simulink model "model"  (R2023a)
settings: Solver=ode4  StartTime=0.0  StopTime=15  FixedStep=0.002  RelTol=1e-3
InitFcn:
  | init;
undefined symbols (not defined in the file): g, N, T, t_f, v_c
libraries: dspsrcs4 x1
settings Model: Creator=Ali  LastModifiedBy=Ali

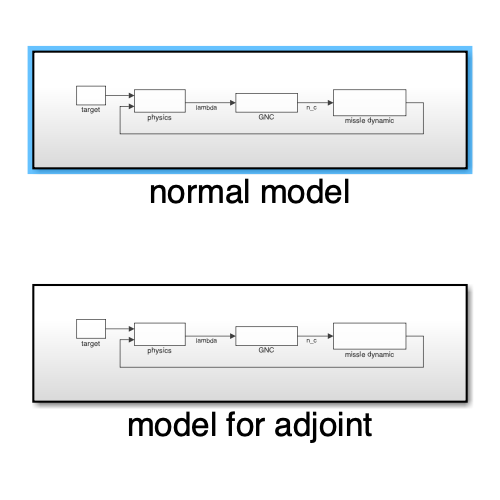
[thumbnail: Simulink's stored preview of the top-level diagram]
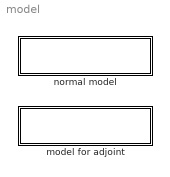
== system model ==
  model for adjoint : Subsystem
  normal model : Subsystem

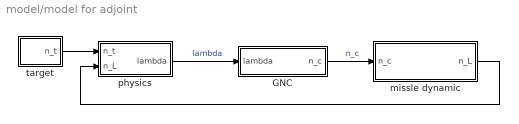
== system model/model for adjoint ==
  GNC : Subsystem
  missle dynamic : Subsystem
  physics : Subsystem
  target : Subsystem
  wires:
  physics/1(lambda) -> GNC/1(lambda)  "lambda"
  target/1(n_t) -> physics/1(n_t)
  GNC/1(n_c) -> missle dynamic/1(n_c)  "n_c"
  missle dynamic/1(n_L) -> physics/2(n_L)

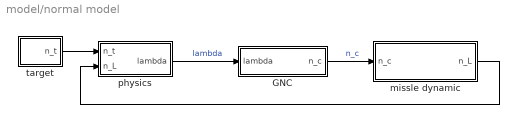
== system model/normal model ==
  GNC : Subsystem
  missle dynamic : Subsystem
  physics : Subsystem
  target : Subsystem
  wires:
  physics/1(lambda) -> GNC/1(lambda)  "lambda"
  target/1(n_t) -> physics/1(n_t)
  GNC/1(n_c) -> missle dynamic/1(n_c)  "n_c"
  missle dynamic/1(n_L) -> physics/2(n_L)

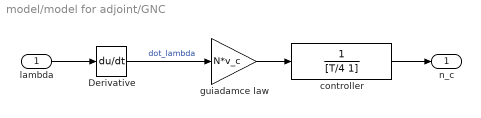
== system model/model for adjoint/GNC ==
  lambda : Inport
  Derivative : Derivative
  controller : TransferFcn  Denominator=[T/4 1]
  guiadamce law : Gain  Gain=N*v_c
  n_c : Outport
  wires:
  guiadamce law/1 -> controller/1
  lambda/1 -> Derivative/1
  Derivative/1 -> guiadamce law/1  "dot_lambda"
  controller/1 -> n_c/1

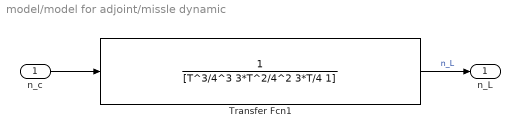
== system model/model for adjoint/missle dynamic ==
  n_c : Inport
  Transfer Fcn1 : TransferFcn  Denominator=[T^3/4^3 3*T^2/4^2 3*T/4 1]
  n_L : Outport
  wires:
  Transfer Fcn1/1 -> n_L/1  "n_L"
  n_c/1 -> Transfer Fcn1/1

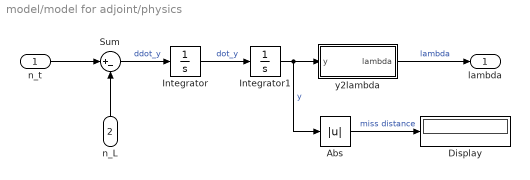
== system model/model for adjoint/physics ==
  n_t : Inport
  n_L : Inport  Port=2
  Abs : Abs  SaturateOnIntegerOverflow=off
  Display : Display
  Integrator : Integrator
  Integrator1 : Integrator
  Sum : Sum  Inputs=|+-
  y2lambda : Subsystem
  lambda : Outport
  wires:
  Sum/1 -> Integrator/1  "ddot_y"
  n_t/1 -> Sum/1
  n_L/1 -> Sum/2
  y2lambda/1(lambda) -> lambda/1  "lambda"
  Integrator/1 -> Integrator1/1  "dot_y"
  Integrator1/1 -> Abs/1, y2lambda/1(y)  "y"
  Abs/1 -> Display/1  "miss distance"

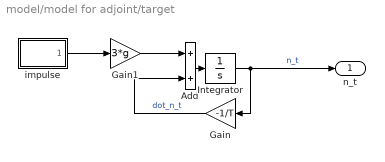
== system model/model for adjoint/target ==
  Add : Sum
  Gain : Gain  Gain=-1/T
  Gain1 : Gain  Gain=3*g
  Integrator : Integrator
  impulse : Subsystem
  n_t : Outport
  wires:
  Gain/1 -> Add/2  "dot_n_t"
  Integrator/1 -> Gain/1, n_t/1  "n_t"
  impulse/1(impulse) -> Gain1/1
  Gain1/1 -> Add/1
  Add/1 -> Integrator/1

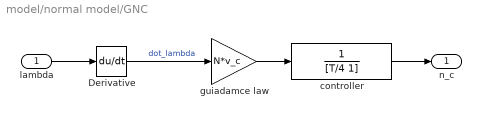
== system model/normal model/GNC ==
  lambda : Inport
  Derivative : Derivative
  controller : TransferFcn  Denominator=[T/4 1]
  guiadamce law : Gain  Gain=N*v_c
  n_c : Outport
  wires:
  guiadamce law/1 -> controller/1
  lambda/1 -> Derivative/1
  Derivative/1 -> guiadamce law/1  "dot_lambda"
  controller/1 -> n_c/1

== system model/normal model/missle dynamic ==
  n_c : Inport
  Transfer Fcn1 : TransferFcn  Denominator=[T^3/4^3 3*T^2/4^2 3*T/4 1]
  n_L : Outport
  wires:
  Transfer Fcn1/1 -> n_L/1  "n_L"
  n_c/1 -> Transfer Fcn1/1

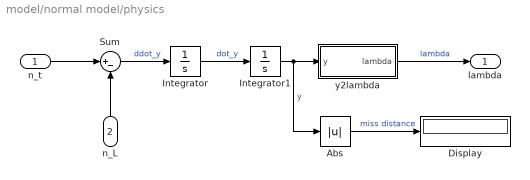
== system model/normal model/physics ==
  n_t : Inport
  n_L : Inport  Port=2
  Abs : Abs  SaturateOnIntegerOverflow=off
  Display : Display
  Integrator : Integrator
  Integrator1 : Integrator
  Sum : Sum  Inputs=|+-
  y2lambda : Subsystem
  lambda : Outport
  wires:
  Sum/1 -> Integrator/1  "ddot_y"
  n_t/1 -> Sum/1
  n_L/1 -> Sum/2
  y2lambda/1(lambda) -> lambda/1  "lambda"
  Integrator/1 -> Integrator1/1  "dot_y"
  Integrator1/1 -> Abs/1, y2lambda/1(y)  "y"
  Abs/1 -> Display/1  "miss distance"

== system model/normal model/target ==
  Gain : Gain  Gain=-1/T
  Integrator : Integrator  InitialCondition=3*g
  n_t : Outport
  wires:
  Gain/1 -> Integrator/1  "dot_n_t"
  Integrator/1 -> n_t/1, Gain/1  "n_t"

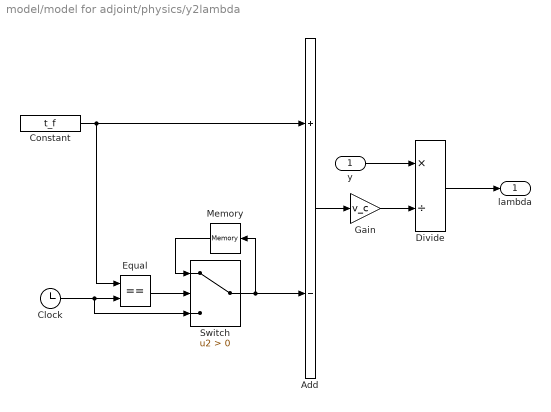
== system model/model for adjoint/physics/y2lambda ==
  y : Inport
  Add : Sum  Inputs=+-
  Clock : Clock
  Constant : Constant  Value=t_f
  Divide : Product  Inputs=*/
  Equal : RelationalOperator  Operator===  OutDataTypeStr=boolean  RndMeth=Simplest  InputSameDT=off
  Gain : Gain  Gain=v_c
  Memory : Memory
  Switch : Switch  Criteria=u2 > Threshold  SaturateOnIntegerOverflow=off  InputSameDT=off
  lambda : Outport
  wires:
  Divide/1 -> lambda/1
  y/1 -> Divide/1
  Gain/1 -> Divide/2
  Constant/1 -> Add/1, Equal/1
  Clock/1 -> Switch/3, Equal/2
  Equal/1 -> Switch/2
  Memory/1 -> Switch/1
  Switch/1 -> Add/2, Memory/1
  Add/1 -> Gain/1

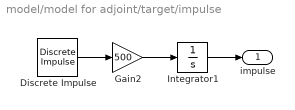
== system model/model for adjoint/target/impulse ==
  Discrete Impulse : dspsrcs4/Discrete  Impulse  Delay=0  SampleTime=0.002  FrameSample=1  OutputFrames=off  dataType=double  isSigned=on  wordLen=16  udDataType=sfix(16)  fracBitsMode=Best precision  numFracBits=15  OutDataTypeStr=double  LastOutDataTypeStr=double
  Gain2 : Gain  Gain=500
  Integrator1 : Integrator
  impulse : Outport
  wires:
  Integrator1/1 -> impulse/1
  Discrete Impulse/1 -> Gain2/1
  Gain2/1 -> Integrator1/1

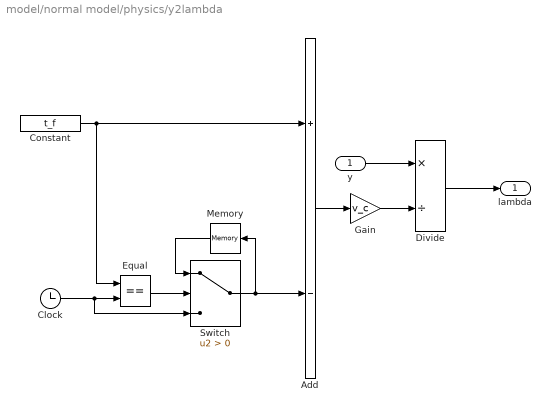
== system model/normal model/physics/y2lambda ==
  y : Inport
  Add : Sum  Inputs=+-
  Clock : Clock
  Constant : Constant  Value=t_f
  Divide : Product  Inputs=*/
  Equal : RelationalOperator  Operator===  OutDataTypeStr=boolean  RndMeth=Simplest  InputSameDT=off
  Gain : Gain  Gain=v_c
  Memory : Memory
  Switch : Switch  Criteria=u2 > Threshold  SaturateOnIntegerOverflow=off  InputSameDT=off
  lambda : Outport
  wires:
  Divide/1 -> lambda/1
  y/1 -> Divide/1
  Gain/1 -> Divide/2
  Constant/1 -> Add/1, Equal/1
  Clock/1 -> Switch/3, Equal/2
  Equal/1 -> Switch/2
  Memory/1 -> Switch/1
  Switch/1 -> Add/2, Memory/1
  Add/1 -> Gain/1
